simulink model "integral_1_pole"  (R2023a)
settings: Solver=VariableStepAuto  StartTime=0.0  StopTime=3  RelTol=1e-3
values from neighbouring files (symbols this model uses):
  A = [a11 a21 a12 a22]    [calc_A.m]    (also in modelo.m = [a11 a12)
  Ad = [-1/t_beta 0 ... (first row only)    [calc_KMax.m]    (also in calc_Kmin.m; modelo.m)
  B = [b11 b21 b12 b22]    [calc_B.m]    (also in calc_inv_B.m = [b11 b12; b21 b22]; modelo.m = [b11 b12)
  C = [1 0 ... (first row only)    [modelo.m]
  D = [0 0;0 0]    [modelo.m]
  E = [e1 e2]    [calc_E.m]    (also in modelo.m = [e1)
  Ed = [k_beta/t_beta ... (first row only)    [calc_KMax.m]    (also in calc_Kmin.m; modelo.m)
  kfb_h2 = [K_H2(1,3),K_H2(1,4);K_H2(2,3),K_H2(2,4)]    [modelo.m]
  kfb_hinf = [K_Hinf(1,3),K_Hinf(1,4);K_Hinf(2,3),K_Hinf(2,4)]    [modelo.m]
  kfb_l1 = [K_L1(1,3),K_L1(1,4);K_L1(2,3),K_L1(2,4)]    [modelo.m]
  kff_h2 = [K_H2(1,1),K_H2(1,2);K_H2(2,1),K_H2(2,2)]    [modelo.m]
  kff_hinf = [K_Hinf(1,1),K_Hinf(1,2);K_Hinf(2,1),K_Hinf(2,2)]    [modelo.m]
  kff_l1 = [K_L1(1,1),K_L1(1,2);K_L1(2,1),K_L1(2,2)]    [modelo.m]
  x0 = [0, 0]    [modelo.m]
undefined symbols (not defined in the file or in its folder): sigbuilder_block
settings Model: Creator=Ferna  LastModifiedBy=Ferna

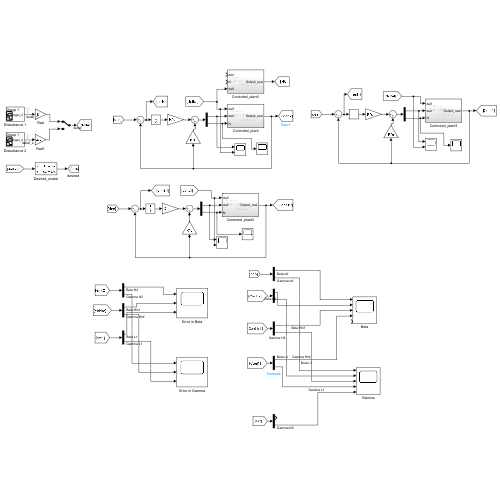
[thumbnail: Simulink's stored preview of the top-level diagram]
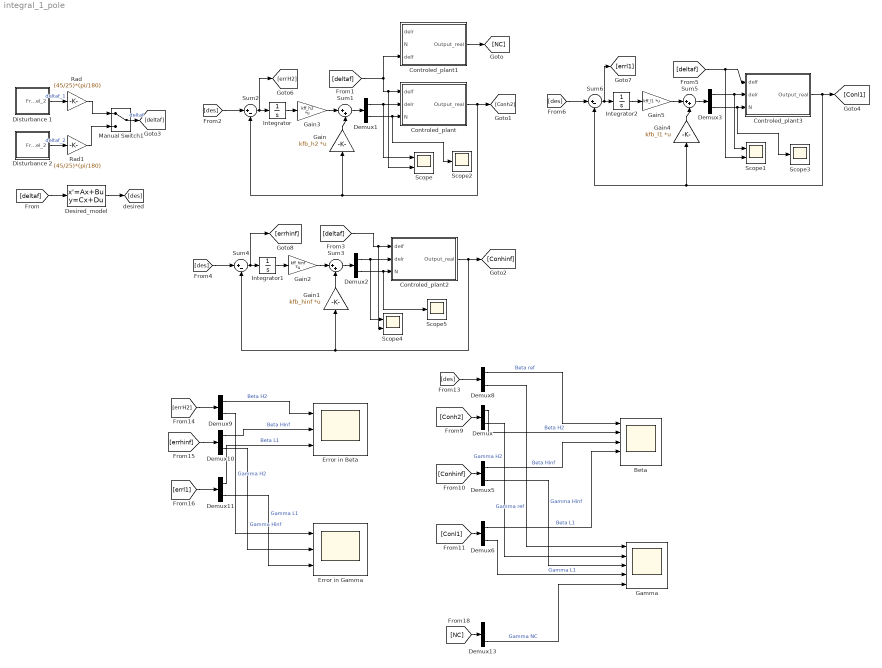
== system integral_1_pole ==
  Beta : Scope  NumInputPorts=5
  Controled_plant : Subsystem
  Controled_plant1 : Subsystem
  Controled_plant2 : Subsystem
  Controled_plant3 : Subsystem
  Demux{,1..3,5..6,8..11,13} (11 alike) : Demux  Outputs=2
  Desired_model : StateSpace  A=Ad  B=Ed  C=[1,0;0,1]  D=zeros(2,1)  InitialCondition=0
  Disturbance 1 : Subsystem  Tag=STV Subsys  LoadFcn=sigbuilder_block('load');  StartFcn=sigbuilder_block('start');  StopFcn=sigbuilder_block('stop');  ClipboardFcn=sigbuilder_block('clipboard');  mask(Sigbuilder block){tuvar=[0:10]}
      mask help: Simulink:masks:SigbuilderBlock_MD
      mask init:
      | if ~strcmp(get_param(bdroot(gcbh),'SimulationStatus'),'stopped') tuvar = sigbuilder_block('maskInit'); end
      settings: CopyFcn=sigbuilder_block('copy');  DeleteFcn=sigbuilder_block('delete');  ModelCloseFcn=sigbuilder_block('modelClose');  PreSaveFcn=sigbuilder_block('preSave');  PauseFcn=sigbuilder_block('pause');  ContinueFcn=sigbuilder_block('continue');  NameChangeFcn=sigbuilder_block('namechange');  OpenFcn=sigbuilder_block('open',[265.8 141.6 550.8 400.2 ]);  CloseFcn=sigbuilder_block('close');
      mask Display: plot(0, 0, 100, 100,[2, 2, 32, 32, 2], [68, 8, 8, 68, 68],[32, 2], [38, 38], [32, 19, 2],[53, 60, 44], [32, 17, 17, 2],[16, 16, 31, 31]);txt = getActiveGroup(gcbh);text(2, 100, txt,'verticalAlignment', 'top');
  Disturbance 2 : Subsystem  Tag=STV Subsys  LoadFcn=sigbuilder_block('load');  StartFcn=sigbuilder_block('start');  StopFcn=sigbuilder_block('stop');  ClipboardFcn=sigbuilder_block('clipboard');  mask(Sigbuilder block){tuvar=[0:10]}
      mask help: Simulink:masks:SigbuilderBlock_MD
      mask init:
      | if ~strcmp(get_param(bdroot(gcbh),'SimulationStatus'),'stopped') tuvar = sigbuilder_block('maskInit'); end
      settings: CopyFcn=sigbuilder_block('copy');  DeleteFcn=sigbuilder_block('delete');  ModelCloseFcn=sigbuilder_block('modelClose');  PreSaveFcn=sigbuilder_block('preSave');  PauseFcn=sigbuilder_block('pause');  ContinueFcn=sigbuilder_block('continue');  NameChangeFcn=sigbuilder_block('namechange');  OpenFcn=sigbuilder_block('open',[265.8 141.6 550.8 400.2 ]);  CloseFcn=sigbuilder_block('close');
      mask Display: plot(0, 0, 100, 100,[2, 2, 32, 32, 2], [68, 8, 8, 68, 68],[32, 2], [38, 38], [32, 19, 2],[53, 60, 44], [32, 17, 17, 2],[16, 16, 31, 31]);txt = getActiveGroup(gcbh);text(2, 100, txt,'verticalAlignment', 'top');
  Error in Beta : Scope  NumInputPorts=3
  Error in Gamma : Scope  NumInputPorts=3
  Gain : Gain  Gain=kfb_h2  Multiplication=Matrix(K*u)
  Gain1 : Gain  Gain=kfb_hinf  Multiplication=Matrix(K*u)
  Gain2 : Gain  Gain=kff_hinf  Multiplication=Matrix(K*u)
  Gain3 : Gain  Gain=kff_h2  Multiplication=Matrix(K*u)
  Gain4 : Gain  Gain=kfb_l1  Multiplication=Matrix(K*u)
  Gain5 : Gain  Gain=kff_l1  Multiplication=Matrix(K*u)
  Gamma : Scope  NumInputPorts=5
  Integrator : Integrator
  Integrator1 : Integrator
  Integrator2 : Integrator
  Manual Switch1 : ManualSwitch
  Rad : Gain  Gain=(45/25)*(pi/180)
  Rad1 : Gain  Gain=(45/25)*(pi/180)
  Scope : Scope  NumInputPorts=2
  Scope1 : Scope  NumInputPorts=2
  Scope2 : Scope
  Scope3 : Scope
  Scope4 : Scope  NumInputPorts=2
  Scope5 : Scope
  Sum1 : Sum  Inputs=|++
  Sum2 : Sum  Inputs=|+-
  Sum3 : Sum  Inputs=|++
  Sum4 : Sum  Inputs=|+-
  Sum5 : Sum  Inputs=|++
  Sum6 : Sum  Inputs=|+-
  wires:
  Gain/1 -> Sum1/2
  Disturbance 1/1(Front steering angel_2) -> Rad/1  "deltaf_1"
  Demux1/1 -> Scope/1, Controled_plant/2(delr)
  Rad/1 -> Manual Switch1/1
  Gain3/1 -> Sum1/1
  Controled_plant1/1(Output_real) -> [NC]
  Rad1/1 -> Manual Switch1/2
  Demux1/2 -> Scope2/1, Controled_plant/3(N)
  Desired_model/1 -> [des]
  Disturbance 2/1(Front steering angel_2) -> Rad1/1  "deltaf_2"
  Sum1/1 -> Demux1/1
  Sum2/1 -> [errH2], Integrator/1
  Integrator/1 -> Gain3/1
  Controled_plant/1(Output_real) -> Gain/1, Sum2/2, [Conh2]
  Manual Switch1/1 -> [deltaf]  "deltaf"
  [deltaf] -> Desired_model/1
  [deltaf] -> Controled_plant1/3(delf), Scope/2, Controled_plant/1(delf)
  [des] -> Sum2/1
  [des] -> Sum4/1
  [deltaf] -> Scope4/2, Controled_plant2/1(delf)
  Controled_plant2/1(Output_real) -> Sum4/2, Gain1/1, [Conhinf]
  Gain1/1 -> Sum3/2
  Demux2/1 -> Controled_plant2/2(delr), Scope4/1
  Sum4/1 -> [errhinf], Integrator1/1
  Integrator1/1 -> Gain2/1
  Demux2/2 -> Scope5/1, Controled_plant2/3(N)
  Gain2/1 -> Sum3/1
  Sum3/1 -> Demux2/1
  Gain5/1 -> Sum5/1
  Sum5/1 -> Demux3/1
  Sum6/1 -> [errl1], Integrator2/1
  Demux3/1 -> Scope1/1, Controled_plant3/2(delr)
  Controled_plant3/1(Output_real) -> Gain4/1, Sum6/2, [Conl1]
  Integrator2/1 -> Gain5/1
  Gain4/1 -> Sum5/2
  [deltaf] -> Scope1/2, Controled_plant3/1(delf)
  Demux3/2 -> Scope3/1, Controled_plant3/3(N)
  [des] -> Sum6/1
  [Conh2] -> Demux/1
  [Conhinf] -> Demux5/1
  [Conl1] -> Demux6/1
  Demux/1 -> Beta/2  "Beta H2"
  Demux5/1 -> Beta/3  "Beta Hinf"
  Demux6/1 -> Beta/4  "Beta L1"
  Demux/2 -> Gamma/2  "Gamma H2"
  Demux5/2 -> Gamma/3  "Gamma Hinf"
  Demux6/2 -> Gamma/4  "Gamma L1"
  [des] -> Demux8/1
  Demux8/2 -> Gamma/1  "Gamma ref"
  [errH2] -> Demux9/1
  [errl1] -> Demux11/1
  Demux9/1 -> Error in Beta/1  "Beta H2"
  Demux10/1 -> Error in Beta/2  "Beta Hinf"
  [errhinf] -> Demux10/1
  Demux11/1 -> Error in Beta/3  "Beta L1"
  Demux9/2 -> Error in Gamma/1  "Gamma H2"
  Demux10/2 -> Error in Gamma/2  "Gamma Hinf"
  Demux11/2 -> Error in Gamma/3  "Gamma L1"
  [NC] -> Demux13/1
  Demux13/2 -> Gamma/5  "Gamma NC"
  Demux8/1 -> Beta/1  "Beta ref"

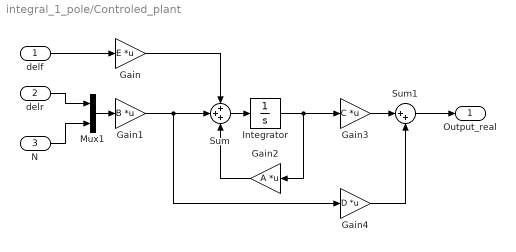
== system integral_1_pole/Controled_plant ==
  delf : Inport
  delr : Inport  Port=2
  N : Inport  Port=3
  Gain : Gain  Gain=E  Multiplication=Matrix(K*u)
  Gain1 : Gain  Gain=B  Multiplication=Matrix(K*u)
  Gain2 : Gain  Gain=A  Multiplication=Matrix(K*u)
  Gain3 : Gain  Gain=C  Multiplication=Matrix(K*u)
  Gain4 : Gain  Gain=D  Multiplication=Matrix(K*u)
  Integrator : Integrator  InitialCondition=x0
  Mux1 : Mux  Inputs=2
  Sum : Sum  Inputs=+++
  Sum1 : Sum  Inputs=|++
  Output_real : Outport
  wires:
  Gain1/1 -> Gain4/1, Sum/2
  Gain4/1 -> Sum1/2
  delr/1 -> Mux1/1
  delf/1 -> Gain/1
  Integrator/1 -> Gain3/1, Gain2/1
  Gain/1 -> Sum/1
  Sum1/1 -> Output_real/1
  Gain3/1 -> Sum1/1
  N/1 -> Mux1/2
  Mux1/1 -> Gain1/1
  Sum/1 -> Integrator/1
  Gain2/1 -> Sum/3

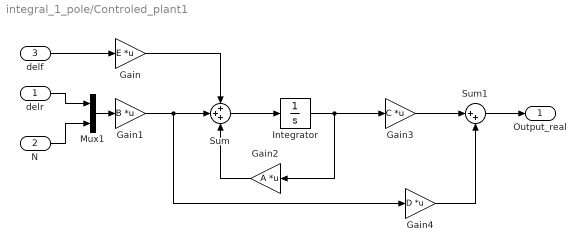
== system integral_1_pole/Controled_plant1 ==
  delr : Inport
  N : Inport  Port=2
  delf : Inport  Port=3
  Gain : Gain  Gain=E  Multiplication=Matrix(K*u)
  Gain1 : Gain  Gain=B  Multiplication=Matrix(K*u)
  Gain2 : Gain  Gain=A  Multiplication=Matrix(K*u)
  Gain3 : Gain  Gain=C  Multiplication=Matrix(K*u)
  Gain4 : Gain  Gain=D  Multiplication=Matrix(K*u)
  Integrator : Integrator  InitialCondition=x0
  Mux1 : Mux  Inputs=2
  Sum : Sum  Inputs=+++
  Sum1 : Sum  Inputs=|++
  Output_real : Outport
  wires:
  Gain2/1 -> Sum/3
  Sum/1 -> Integrator/1
  Mux1/1 -> Gain1/1
  N/1 -> Mux1/2
  Gain3/1 -> Sum1/1
  Sum1/1 -> Output_real/1
  Gain/1 -> Sum/1
  Integrator/1 -> Gain2/1, Gain3/1
  delf/1 -> Gain/1
  delr/1 -> Mux1/1
  Gain4/1 -> Sum1/2
  Gain1/1 -> Sum/2, Gain4/1

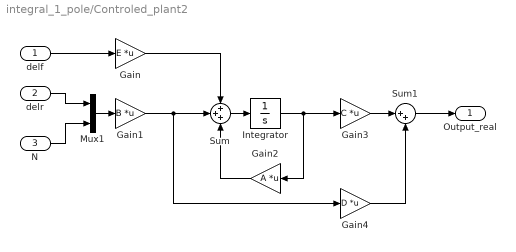
== system integral_1_pole/Controled_plant2 ==
  delf : Inport
  delr : Inport  Port=2
  N : Inport  Port=3
  Gain : Gain  Gain=E  Multiplication=Matrix(K*u)
  Gain1 : Gain  Gain=B  Multiplication=Matrix(K*u)
  Gain2 : Gain  Gain=A  Multiplication=Matrix(K*u)
  Gain3 : Gain  Gain=C  Multiplication=Matrix(K*u)
  Gain4 : Gain  Gain=D  Multiplication=Matrix(K*u)
  Integrator : Integrator  InitialCondition=x0
  Mux1 : Mux  Inputs=2
  Sum : Sum  Inputs=+++
  Sum1 : Sum  Inputs=|++
  Output_real : Outport
  wires:
  Gain1/1 -> Gain4/1, Sum/2
  Gain4/1 -> Sum1/2
  delr/1 -> Mux1/1
  delf/1 -> Gain/1
  Integrator/1 -> Gain3/1, Gain2/1
  Gain/1 -> Sum/1
  Sum1/1 -> Output_real/1
  Gain3/1 -> Sum1/1
  N/1 -> Mux1/2
  Mux1/1 -> Gain1/1
  Sum/1 -> Integrator/1
  Gain2/1 -> Sum/3

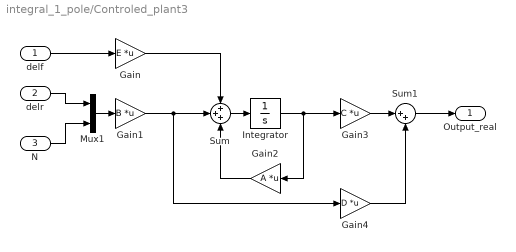
== system integral_1_pole/Controled_plant3 ==
  delf : Inport
  delr : Inport  Port=2
  N : Inport  Port=3
  Gain : Gain  Gain=E  Multiplication=Matrix(K*u)
  Gain1 : Gain  Gain=B  Multiplication=Matrix(K*u)
  Gain2 : Gain  Gain=A  Multiplication=Matrix(K*u)
  Gain3 : Gain  Gain=C  Multiplication=Matrix(K*u)
  Gain4 : Gain  Gain=D  Multiplication=Matrix(K*u)
  Integrator : Integrator  InitialCondition=x0
  Mux1 : Mux  Inputs=2
  Sum : Sum  Inputs=+++
  Sum1 : Sum  Inputs=|++
  Output_real : Outport
  wires:
  Gain1/1 -> Gain4/1, Sum/2
  Gain4/1 -> Sum1/2
  delr/1 -> Mux1/1
  delf/1 -> Gain/1
  Integrator/1 -> Gain3/1, Gain2/1
  Gain/1 -> Sum/1
  Sum1/1 -> Output_real/1
  Gain3/1 -> Sum1/1
  N/1 -> Mux1/2
  Mux1/1 -> Gain1/1
  Sum/1 -> Integrator/1
  Gain2/1 -> Sum/3

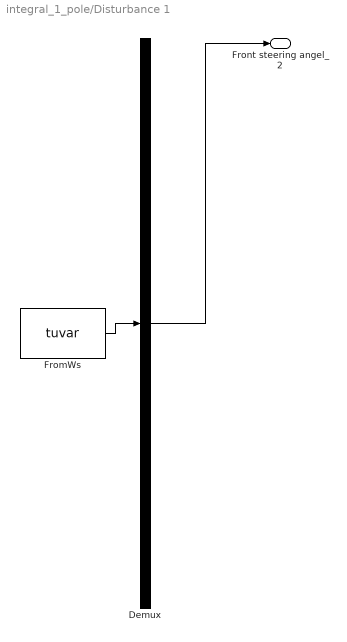
== system integral_1_pole/Disturbance 1 ==
  Demux : Demux  Tag=STV Demux  Outputs=1
      settings: DisplayOption=none
  FromWs : FromWorkspace  Tag=STV FromWs  VariableName=tuvar
      SigBuilderData=|
      | common.afterFinalStr = 'Extrapolate'
      | common.sampleTime = 0
      | dataSet.timeRange = [0 3]
      | dataSet.name = 'Group 1'
      | sbobj.Groups.Name = 'Group 1'
      | sbobj.Groups.Signals.Name = 'Front steering angel_2'
      | sbobj.Groups.Signals.XData = [0 0.5 1 1.5 2 2.5 3]
      | sbobj.Groups.Signals.YData = [-0.005 0.005 1 1 0 0 0]
      | sbobj.Groups.TimeRange = [0 3]
  Front steering angel_2 : Outport  Tag=STV Outport
  wires:
  FromWs/1 -> Demux/1
  Demux/1 -> Front steering angel_2/1

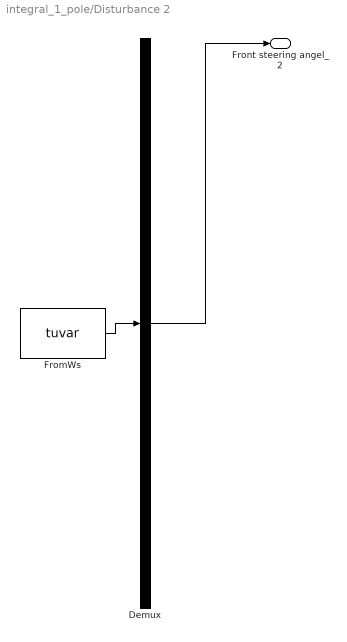
== system integral_1_pole/Disturbance 2 ==
  Demux : Demux  Tag=STV Demux  Outputs=1
      settings: DisplayOption=none
  FromWs : FromWorkspace  Tag=STV FromWs  VariableName=tuvar
      SigBuilderData=|
      | common.afterFinalStr = 'Extrapolate'
      | common.sampleTime = 0
      | dataSet.timeRange = [0 3]
      | dataSet.name = 'Group 1'
      | sbobj.Groups.Name = 'Group 1'
      | sbobj.Groups.Signals.Name = 'Front steering angel_2'
      | sbobj.Groups.Signals.XData = [0 0.187490625469 0.374981250937 0.562471876406 0.749962501875 0.937453127344 1.12494375281 1.31243437828 1.49992500375 1.68741562922 1.87490625469 2.06239688016 2.24988750562 2.43737813109 2.62486875656 2.81235938203 2.9998500075 3]
      | sbobj.Groups.Signals.YData = [0 0.565685424949 0.8 0.565685424949 9.79717439318e-17 -0.565685424949 -0.8 -0.565685424949 0 0 0 0 0 0 0 0 0 0]
      | sbobj.Groups.TimeRange = [0 3]
  Front steering angel_2 : Outport  Tag=STV Outport
  wires:
  Demux/1 -> Front steering angel_2/1
  FromWs/1 -> Demux/1
